simulink model "Model2"  (R2019b)
settings: Solver=VariableStepAuto  StartTime=0.0  StopTime=4  MaxStep=1e-3  RelTol=1e-3
undefined symbols (not defined in the file): fsin, ftr, k
libraries: simulink x1
settings Model: Creator=atmat  LastModifiedBy=atmat

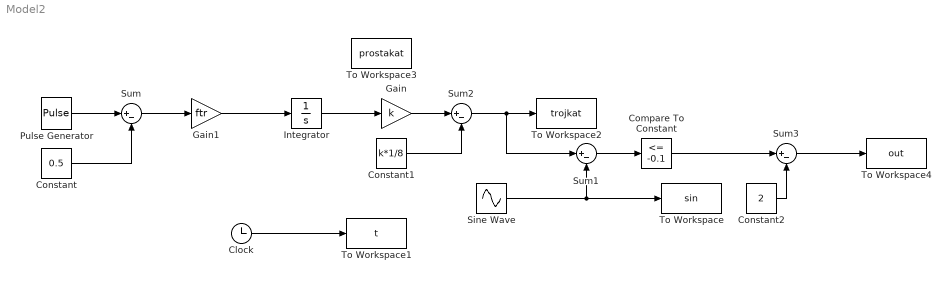
== system Model2 ==
  Clock : Clock
  Compare To Constant : simulink/Logic and Bit Operations/Compare To Constant  relop=<=  const=-0.1  OutDataTypeStr=boolean
  Constant : Constant  Value=0.5
  Constant1 : Constant  Value=k*1/8
  Constant2 : Constant  Value=2
  Gain : Gain  Gain=k
  Gain1 : Gain  Gain=ftr
  Integrator : Integrator
  Pulse Generator : DiscretePulseGenerator  PulseType=Time based  Period=1/ftr  PulseWidth=50
  Sine Wave : Sin  Frequency=fsin*(pi)  SampleTime=0
  Sum{,1..3} (4 alike) : Sum  Inputs=|+-
  To Workspace : ToWorkspace  VariableName=sin  SampleTime=-1
  To Workspace1 : ToWorkspace  VariableName=t  SampleTime=-1
  To Workspace2 : ToWorkspace  VariableName=trojkat  SampleTime=-1
  To Workspace3 : ToWorkspace  VariableName=prostakat  SampleTime=-1
  To Workspace4 : ToWorkspace  VariableName=out  SampleTime=-1
  wires:
  Pulse Generator/1 -> Sum/1
  Constant/1 -> Sum/2
  Integrator/1 -> Gain/1
  Sum1/1 -> Compare To Constant/1
  Gain/1 -> Sum2/1
  Sum2/1 -> Sum1/1, To Workspace2/1
  Constant1/1 -> Sum2/2
  Gain1/1 -> Integrator/1
  Sum/1 -> Gain1/1
  Sine Wave/1 -> To Workspace/1, Sum1/2
  Clock/1 -> To Workspace1/1
  Constant2/1 -> Sum3/2
  Compare To Constant/1 -> Sum3/1
  Sum3/1 -> To Workspace4/1
